simulink model "Adapive PID Controller for BLDC Speed Control"  (R2018a)
settings: Solver=ode45  StartTime=0  StopTime=0.4  FixedStep=Ts  MaxStep=1e-3  RelTol=1e-3  AbsTol=1e-3  EnableMultiTasking=on
InitFcn:
  | c_boost = 2200e-006;
  | f_nom = 50;
  | k_Idc = 3;
  | k_Vin = 40.6586;
  | k_Vref = 0.03;
  | k_Vdc = 0.03;
  | l_boost = 0.006;
  | l_filter = 50E-006;
  | r_boost = 1e-003;
  | r_line = 1;
  | r_load = .04E003;
  | S_ref = 3000;
  | v_nom = 220;
undefined symbols (not defined in the file): sigbuilder_block
libraries: simulink x6, powerlib x4, dspstat3 x1
Description:
  | This demonstration illustrates use of the BLDC in a closed-loop
  | speed and voltage control on a 1 kW, 3000 rpm industrial motor
settings Model: ExtModeAutoUpdateStatusClock=off  Creator=Olivier Tremblay  LastModifiedBy=Mehdi
settings SolverCC: AutoScaleAbsTol=off
settings DataIOCC: LimitDataPoints=on  SaveFormat=Array  SignalLoggingSaveFormat=ModelDataLogs  SignalLoggingName=sigsOut
settings OptimizationCC: ExpressionDepthLimit=2147483647  InitFltsAndDblsToZero=on  LifeSpan=inf
settings DebuggingCC: SaveWithParameterizedLinksMsg=none  UnderspecifiedInitializationDetection=Classic  MergeDetectMultiDrivingBlocksExec=none  SignalResolutionControl=TryResolveAllWithWarning  MultiTaskDSMMsg=warning  MultiTaskCondExecSysMsg=none  SigSpecEnsureSampleTimeMsg=none  FcnCallInpInsideContextMsg=warning  RootOutportRequireBusObject=none  StateNameClashWarn=warning  SFUnexpectedBacktrackingDiag=warning  SFNoUnconditionalDefaultTransitionDiag=warning  SFExecutionAtInitializationDiag=none
settings HardwareCC: ProdBitPerPointer=32  ProdBitPerSizeT=32  ProdBitPerPtrDiffT=32  ProdLargestAtomicFloat=None  ProdIntDivRoundTo=Undefined  ProdEndianess=Unspecified  ProdWordSize=32  ProdHWDeviceType=32-bit Generic  TargetUnknown=on
settings ModelReferenceCC: PropagateSignalLabelsOutOfModel=off
settings CodeAppCC: StateflowObjectComments=on
settings GRTTargetCC: TargetFcnLib=ansi_tfl_tmw.mat  TargetLangStandard=C89/C90 (ANSI)  GeneratePreprocessorConditionals=Disable all  CombineOutputUpdateFcns=off  GRTInterface=on
settings ConfigComp: CovMetricSettings=dw  CovHtmlReporting=on  CovSaveCumulativeToWorkspaceVar=on  CovSaveSingleToWorkspaceVar=on  CovExternalEMLEnable=off
settings SimscapeCC: SimscapeNormalizeSystem=off

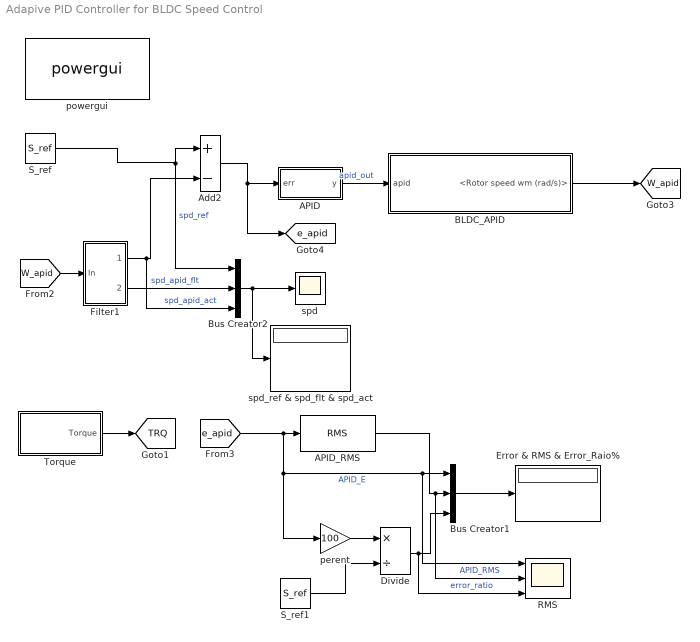
== system Adapive PID Controller for BLDC Speed Control ==
  APID : Subsystem
  APID_RMS : dspstat3/RMS  run=on  directionMode=Each column  dimension=1  InputProcessing=Columns as channels (frame based)  reset_popup=None
  Add2 : Sum  Inputs=|+-
  BLDC_APID : Subsystem
  Bus Creator1 : BusCreator  Inputs=3
  Bus Creator2 : BusCreator  Inputs=3
  Divide : Product  Inputs=*/
  Error & RMS & Error_Raio% : Display
  Filter1 : Subsystem
  RMS : Scope  NumInputPorts=3
  S_ref : Constant  Value=S_ref
  S_ref1 : Constant  Value=S_ref
  Torque : Subsystem  Tag=STV Subsys  LoadFcn=sigbuilder_block('load');  StartFcn=sigbuilder_block('start');  StopFcn=sigbuilder_block('stop');  ClipboardFcn=sigbuilder_block('clipboard');  mask(Sigbuilder block){tuvar=[0:10]}
      mask help: Simulink:masks:SigbuilderBlock_MD
      mask init:
      | if ~strcmp(get_param(bdroot(gcbh),'SimulationStatus'),'stopped') tuvar = sigbuilder_block('maskInit'); end
      settings: CopyFcn=sigbuilder_block('copy');  DeleteFcn=sigbuilder_block('delete');  ModelCloseFcn=sigbuilder_block('modelClose');  PreSaveFcn=sigbuilder_block('preSave');  PauseFcn=sigbuilder_block('pause');  ContinueFcn=sigbuilder_block('continue');  NameChangeFcn=sigbuilder_block('namechange');  OpenFcn=sigbuilder_block('open',[46.5 196.5 1012.5 447.75 ]);  CloseFcn=sigbuilder_block('close');
      mask Display: plot(0, 0, 100, 100,[2, 2, 32, 32, 2], [68, 8, 8, 68, 68],[32, 2], [38, 38], [32, 19, 2],[53, 60, 44], [32, 17, 17, 2],[16, 16, 31, 31]);txt = getActiveGroup(gcbh);text(2, 100, txt,'verticalAlignment', 'top');
  perent : Gain  Gain=100
  powergui : powerlib/powergui  SimulationMode=Discrete  SampleTime=1e-6  frequency=60  Iterations=50  frequencyindice=0  Pbase=100e6  ErrMax=1e-4  UnitsV=kV  UnitsW=MW  buscounter=0  FunctionMessages=off  echomessages=off  EnableUseOfTLC=off  CurrentSourceSwitches=off  DisableSnubberDevices=off  DisableRonSwitches=off  DisableVfSwitches=off  DisplayEquations=off  SolverType=Tustin  Interpol=off  ExternalGateDelay=off  methode=off  Ts=0  x0status=blocks  SPID=off  SwTol=0  HookPort=off  RestoreLinks=warning  ResistiveCurrentMeasurement=off  Frange=[0:2:500]  Ylog=off  Xlog=on  ShowGrid=off  save=off  variable=ZData  structure=ScopeData7  ZoomFFT=off  StartTime=0.24  cycles=1  DisplayStyle=1  fundamental=50  FreqAxis=on  MaxFrequency=1000  frequencyindicesteady=1  RmsSteady=1  display=off
  spd : Scope
  spd_ref & spd_flt & spd_act : Display
  tag scope: TRQ=global, W_apid=global, e_apid=global
  wires:
  S_ref/1 -> Bus Creator2/1, Add2/1  "spd_ref"
  Torque/1(Torque) -> [TRQ]
  BLDC_APID/1(<Rotor speed wm (rad/s)>) -> [W_apid]
  APID/1(y) -> BLDC_APID/1(apid)  "apid_out"
  Add2/1 -> APID/1(err), [e_apid]
  Filter1/1(sp_fb) -> Bus Creator2/3, Add2/2  "spd_apid_act"
  [W_apid] -> Filter1/1(In)
  Filter1/2(sp_fl) -> Bus Creator2/2  "spd_apid_flt"
  Bus Creator2/1 -> spd_ref & spd_flt & spd_act/1, spd/1
  APID_RMS/1 -> RMS/2, Bus Creator1/2  "APID_RMS"
  [e_apid] -> perent/1, RMS/1, Bus Creator1/1, APID_RMS/1  "APID_E"
  Bus Creator1/1 -> Error & RMS & Error_Raio%/1
  S_ref1/1 -> Divide/2
  Divide/1 -> RMS/3, Bus Creator1/3  "error_ratio"
  perent/1 -> Divide/1

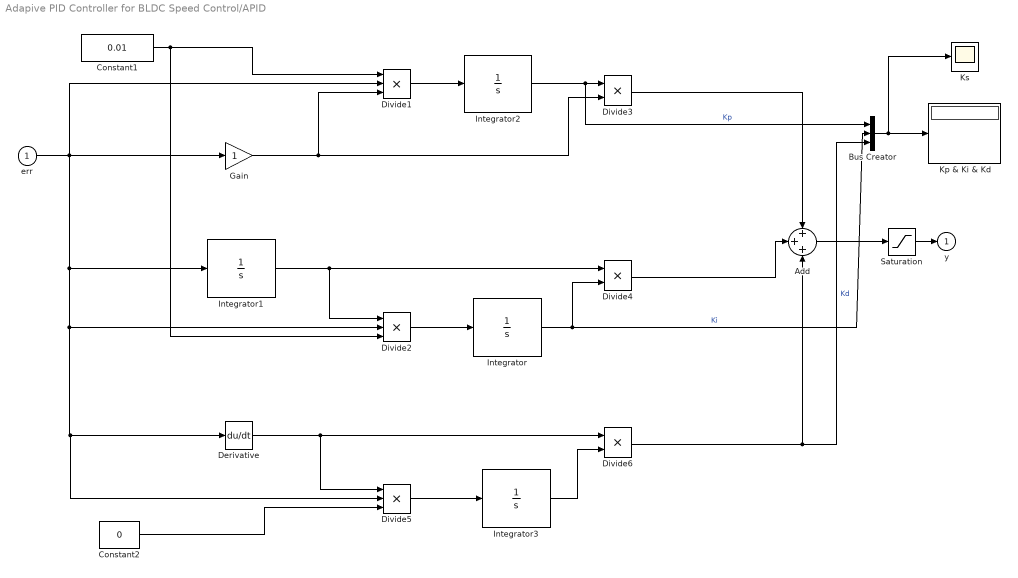
== system Adapive PID Controller for BLDC Speed Control/APID ==
  err : Inport
  Add : Sum  Inputs=+++
  Bus Creator : BusCreator  Inputs=3
  Constant1 : Constant  Value=0.01
  Constant2 : Constant  Value=0
  Derivative : Derivative  CoefficientInTFapproximation=0
  Divide1 : Product  Inputs=***
  Divide2 : Product  Inputs=***
  Divide3 : Product  Inputs=**
  Divide4 : Product  Inputs=**
  Divide5 : Product  Inputs=***
  Divide6 : Product  Inputs=**
  Gain : Gain
  Integrator : Integrator  ZeroCross=off
  Integrator1 : Integrator  InitialCondition=-2  ZeroCross=off
  Integrator2 : Integrator  ZeroCross=off
  Integrator3 : Integrator  ZeroCross=off
  Kp & Ki & Kd : Display
  Ks : Scope
  Saturation : Saturate  UpperLimit=1000  LowerLimit=-1000
  y : Outport  InitialOutput=0
  wires:
  Add/1 -> Saturation/1
  err/1 -> Divide1/2, Derivative/1, Divide5/2, Divide2/2, Integrator1/1, Gain/1
  Gain/1 -> Divide3/2, Divide1/3
  Integrator1/1 -> Divide4/1, Divide2/1
  Divide2/1 -> Integrator/1
  Divide1/1 -> Integrator2/1
  Integrator2/1 -> Bus Creator/1, Divide3/1  "Kp"
  Integrator/1 -> Bus Creator/2, Divide4/2  "Ki"
  Divide3/1 -> Add/1
  Divide4/1 -> Add/2
  Constant1/1 -> Divide2/3, Divide1/1
  Derivative/1 -> Divide5/1, Divide6/1
  Divide5/1 -> Integrator3/1
  Integrator3/1 -> Divide6/2
  Divide6/1 -> Bus Creator/3, Add/3  "Kd"
  Constant2/1 -> Divide5/3
  Bus Creator/1 -> Ks/1, Kp & Ki & Kd/1
  Saturation/1 -> y/1

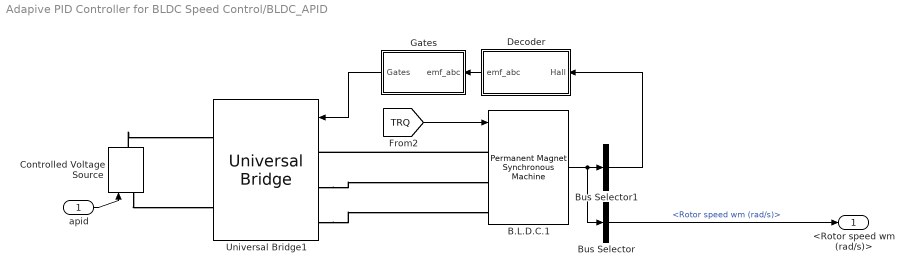
== system Adapive PID Controller for BLDC Speed Control/BLDC_APID ==
  apid : Inport
  B.L.D.C.1 : powerlib/Machines/Permanent Magnet Synchronous Machine  NbPhases=3  FluxDistribution=Trapezoidal  RotorType=Round  MechanicalLoad=Torque Tm  PresetModel=No  ShowDetailedParameters=on  MeasurementBus=off  Resistance=2.8750  Inductance=8.5e-3  dqInductances=[8.5e-3, 8.5e-3]  La=0.000835  MachineConstant=Torque Constant (N.m / A_peak)  Flux=0.175  VoltageCst=146.6077  TorqueCst=1.4  Flat=120  Mechanical="[ 0.8e-3, 1e-3,  4 ]"  PolePairs=4  InitialConditions=[0,0, 0,0]  InitialConditions5ph=[0 0 0 0 0 0]  TsPowergui=0  TsBlock=-1  RefAngle=90 degrees behind phase A axis (modified Park)
      settings: SourceProductName=Simscape Power Systems
  Bus Selector : BusSelector  OutputSignals=Rotor speed wm (rad/s)
  Bus Selector1 : BusSelector  OutputSignals=Hall effect signal h_a,Hall effect signal h_b,Hall effect signal h_c  OutputAsBus=on
  Controlled Voltage Source : powerlib/Electrical Sources/Controlled Voltage Source  Initialize=on  Source_Type=AC  Amplitude=0  Phase=0  Frequency=0  Measurements=None
  Decoder : Subsystem
  Gates : Subsystem
  Universal Bridge1 : powerlib/Power Electronics/Universal Bridge  Arms=3  SnubberResistance=5000  SnubberCapacitance=1e-6  Device=MOSFET / Diodes  Ron=1e-3  Lon=0  ForwardVoltages="[  0  0  ]"  ForwardVoltage=0  GTOparameters=[ 10e-6 , 20e-6 ]  IGBTparameters=[ 1e-6 , 2e-6 ]  Measurements=None  Measurements_2=None  converterType=Rectifier
  <Rotor speed wm (rad/s)> : Outport
  wires:
  apid/1 -> Controlled Voltage Source/1
  Bus Selector/1 -> <Rotor speed wm (rad/s)>/1  "<Rotor speed wm (rad/s)>"
  Gates/1(Gates) -> Universal Bridge1/1
  B.L.D.C.1/1 -> Bus Selector1/1, Bus Selector/1
  Bus Selector1/1 -> Decoder/1("Hall ")
  Decoder/1(emf_abc) -> Gates/1("emf_abc ")
  [TRQ] -> B.L.D.C.1/1
  connections:
  Controlled Voltage Source/LConn1 -- Universal Bridge1/RConn2
  Universal Bridge1/LConn3 -- B.L.D.C.1/LConn3
  Universal Bridge1/LConn2 -- B.L.D.C.1/LConn2
  Controlled Voltage Source/RConn1 -- Universal Bridge1/RConn1
  B.L.D.C.1/LConn1 -- Universal Bridge1/LConn1

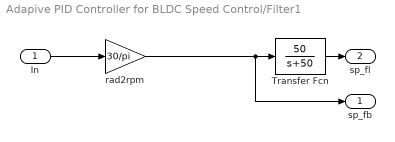
== system Adapive PID Controller for BLDC Speed Control/Filter1 ==
  In : Inport
  Transfer Fcn : TransferFcn  Numerator=[50]  Denominator=[1 50]
  rad2rpm : Gain  Gain=30/pi
  sp_fb : Outport
  sp_fl : Outport  Port=2
  wires:
  rad2rpm/1 -> sp_fb/1, Transfer Fcn/1
  Transfer Fcn/1 -> sp_fl/1
  In/1 -> rad2rpm/1

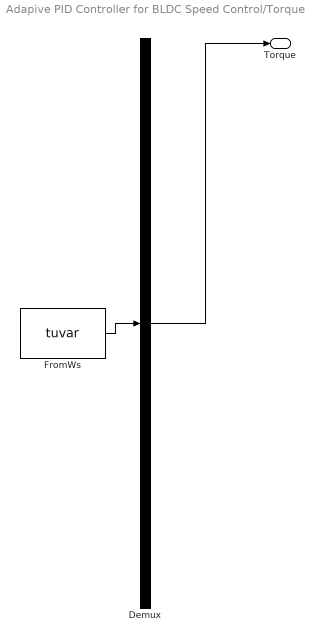
== system Adapive PID Controller for BLDC Speed Control/Torque ==
  Demux : Demux  Tag=STV Demux  Outputs=1
  FromWs : FromWorkspace  Tag=STV FromWs  VariableName=tuvar  SampleTime=0
      SigBuilderData=|
      | common.afterFinalStr = 'Extrapolate'
      | common.sampleTime = 0
      | dataSet.timeRange = [0 10]
      | dataSet.name = 'BLDC Torque'
      | sbobj.Groups.Name = 'BLDC Torque'
      | sbobj.Groups.Signals.Name = 'Torque'
      | sbobj.Groups.Signals.XData = [0 0.2 0.2 10]
      | sbobj.Groups.Signals.YData = [0 0 10 10]
  Torque : Outport  Tag=STV Outport
  wires:
  Demux/1 -> Torque/1
  FromWs/1 -> Demux/1

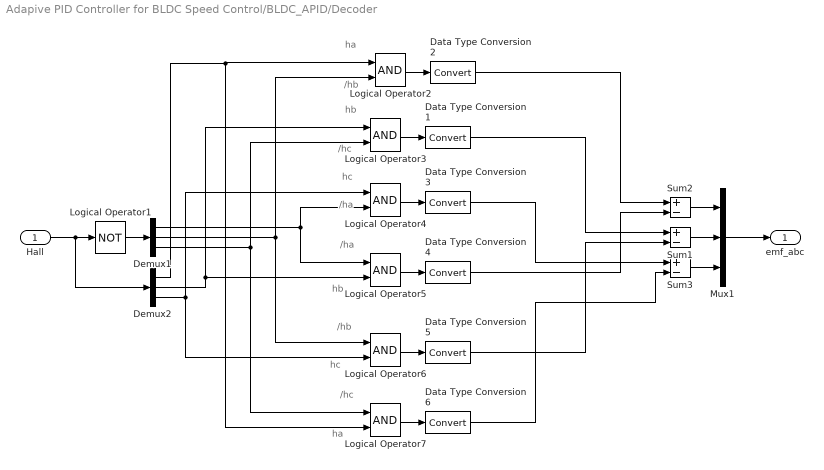
== system Adapive PID Controller for BLDC Speed Control/BLDC_APID/Decoder ==
  note: ha
  note: /hc
  note: hc
  note: /hb
  note: hb
  note: /ha
  note: /ha
  note: hc
  note: /hc
  note: hb
  note: /hb
  note: ha
  "Hall " : Inport
  Data Type Conversion{1..6} (6 alike) : DataTypeConversion
  Demux1 : Demux  Outputs=3
  Demux2 : Demux  Outputs=3
  Logical Operator1 : Logic  Operator=NOT  AllPortsSameDT=off  OutDataTypeStr=boolean
  Logical Operator{2..7} (6 alike) : Logic  AllPortsSameDT=off  OutDataTypeStr=boolean
  Mux1 : Mux  Inputs=3
  Sum1 : Sum  Inputs=+-  OutDataTypeStr=double
  Sum2 : Sum  Inputs=+-  OutDataTypeStr=double
  Sum3 : Sum  Inputs=+-  OutDataTypeStr=double
  emf_abc : Outport
  wires:
  Data Type Conversion6/1 -> Sum3/2
  Data Type Conversion3/1 -> Sum3/1
  Data Type Conversion5/1 -> Sum1/2
  Data Type Conversion1/1 -> Sum1/1
  Data Type Conversion4/1 -> Sum2/2
  Data Type Conversion2/1 -> Sum2/1
  Logical Operator7/1 -> Data Type Conversion6/1
  Logical Operator6/1 -> Data Type Conversion5/1
  Logical Operator5/1 -> Data Type Conversion4/1
  Logical Operator4/1 -> Data Type Conversion3/1
  Logical Operator3/1 -> Data Type Conversion1/1
  Mux1/1 -> emf_abc/1
  Sum3/1 -> Mux1/3
  Sum1/1 -> Mux1/2
  Sum2/1 -> Mux1/1
  Logical Operator2/1 -> Data Type Conversion2/1
  Demux1/1 -> Logical Operator5/1, Logical Operator4/2
  Demux1/2 -> Logical Operator6/1, Logical Operator2/2
  Demux1/3 -> Logical Operator7/1, Logical Operator3/2
  Demux2/1 -> Logical Operator7/2, Logical Operator2/1
  Demux2/2 -> Logical Operator5/2, Logical Operator3/1
  Demux2/3 -> Logical Operator6/2, Logical Operator4/1
  Logical Operator1/1 -> Demux1/1
  "Hall "/1 -> Demux2/1, Logical Operator1/1

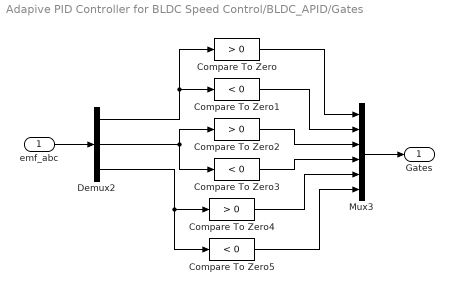
== system Adapive PID Controller for BLDC Speed Control/BLDC_APID/Gates ==
  "emf_abc " : Inport
  Compare To Zero : simulink/Logic and Bit Operations/Compare To Zero  relop=>  OutDataTypeStr=boolean  ZeroCross=off
  Compare To Zero1 : simulink/Logic and Bit Operations/Compare To Zero  relop=<  OutDataTypeStr=boolean  ZeroCross=off
  Compare To Zero2 : simulink/Logic and Bit Operations/Compare To Zero  relop=>  OutDataTypeStr=boolean  ZeroCross=off
  Compare To Zero3 : simulink/Logic and Bit Operations/Compare To Zero  relop=<  OutDataTypeStr=boolean  ZeroCross=off
  Compare To Zero4 : simulink/Logic and Bit Operations/Compare To Zero  relop=>  OutDataTypeStr=boolean  ZeroCross=off
  Compare To Zero5 : simulink/Logic and Bit Operations/Compare To Zero  relop=<  OutDataTypeStr=boolean  ZeroCross=off
  Demux2 : Demux  Outputs=3
  Mux3 : Mux  Inputs=6
  Gates : Outport
  wires:
  Compare To Zero5/1 -> Mux3/6
  Compare To Zero4/1 -> Mux3/5
  Compare To Zero3/1 -> Mux3/4
  Compare To Zero2/1 -> Mux3/3
  Compare To Zero1/1 -> Mux3/2
  Compare To Zero/1 -> Mux3/1
  Demux2/3 -> Compare To Zero5/1, Compare To Zero4/1
  Demux2/2 -> Compare To Zero3/1, Compare To Zero2/1
  Demux2/1 -> Compare To Zero1/1, Compare To Zero/1
  Mux3/1 -> Gates/1
  "emf_abc "/1 -> Demux2/1
